simulink model "MPC_MG_raw_ver1"  (R2021b)
settings: Solver=ode23tb  StartTime=0.0  StopTime=1  RelTol=1e-3
model workspace (MAT data in the model file):
  Ts : Simulink.Parameter (value not decoded)
  secondary_on : Simulink.Parameter (value not decoded)
values from neighbouring files (symbols this model uses):
  A = zeros(4,4)    [MPC_MG_script_raw_dmpc.m]    (also in MPG_MG_July.m = [0 1 1 1; 1 0 0 0; 1 0 0 0; 1 0 0 0]; MPG_MG_freq_script.m = ones(4) - eye(4); Script.m = [0 1 1 1 ; 1 0 1 1 ; 1 1 0 1 ; 1 1 1 0])
  a12 = 0    [Four_DG_MG_PrimaryOnlyScript.m]    (also in MPC_MG_script_raw_dmpc.m; MPC_MG_secondary_script.m)
  a14 = 0    [Four_DG_MG_PrimaryOnlyScript.m]    (also in MPC_MG_script_raw_dmpc.m; MPC_MG_secondary_script.m)
  a21 = 1    [Four_DG_MG_PrimaryOnlyScript.m]    (also in MPC_MG_script_raw_dmpc.m; MPC_MG_secondary_script.m)
  a23 = 0    [Four_DG_MG_PrimaryOnlyScript.m]    (also in MPC_MG_script_raw_dmpc.m; MPC_MG_secondary_script.m)
  a32 = 1    [Four_DG_MG_PrimaryOnlyScript.m]    (also in MPC_MG_script_raw_dmpc.m; MPC_MG_secondary_script.m)
  a34 = 0    [Four_DG_MG_PrimaryOnlyScript.m]    (also in MPC_MG_script_raw_dmpc.m; MPC_MG_secondary_script.m)
  a41 = 1    [Four_DG_MG_PrimaryOnlyScript.m]    (also in MPC_MG_script_raw_dmpc.m; MPC_MG_secondary_script.m)
  a43 = 0    [Four_DG_MG_PrimaryOnlyScript.m]    (also in MPC_MG_script_raw_dmpc.m; MPC_MG_secondary_script.m)
  b1v = 1    [Four_DG_MG_PrimaryOnlyScript.m]    (also in MPC_MG_script_raw_dmpc.m; MPC_MG_secondary_script.m; MPG_MG_July.m; MPG_MG_freq_script.m)
  b1w = 1    [Four_DG_MG_PrimaryOnlyScript.m]    (also in MPC_MG_script_raw_dmpc.m; MPC_MG_secondary_script.m; MPG_MG_July.m; MPG_MG_freq_script.m)
  b2v = 0    [Four_DG_MG_PrimaryOnlyScript.m]    (also in MPC_MG_script_raw_dmpc.m; MPC_MG_secondary_script.m; MPG_MG_July.m; MPG_MG_freq_script.m)
  b2w = 0    [Four_DG_MG_PrimaryOnlyScript.m]    (also in MPC_MG_script_raw_dmpc.m; MPC_MG_secondary_script.m; MPG_MG_July.m; MPG_MG_freq_script.m)
  b3v = 0    [Four_DG_MG_PrimaryOnlyScript.m]    (also in MPC_MG_script_raw_dmpc.m; MPC_MG_secondary_script.m; MPG_MG_July.m; MPG_MG_freq_script.m)
  b3w = 0    [Four_DG_MG_PrimaryOnlyScript.m]    (also in MPC_MG_script_raw_dmpc.m; MPC_MG_secondary_script.m; MPG_MG_July.m; MPG_MG_freq_script.m)
  b4v = 0    [Four_DG_MG_PrimaryOnlyScript.m]    (also in MPC_MG_script_raw_dmpc.m; MPC_MG_secondary_script.m; MPG_MG_July.m; MPG_MG_freq_script.m)
  b4w = 0    [Four_DG_MG_PrimaryOnlyScript.m]    (also in MPC_MG_script_raw_dmpc.m; MPC_MG_secondary_script.m; MPG_MG_July.m; MPG_MG_freq_script.m)
  C_f = 50e-6    (= 5e-05)    [Four_DG_MG_PrimaryOnlyScript.m]    (also in MPC_MG_script.m; MPC_MG_script_raw_dmpc.m; MPC_MG_secondary_script.m; MPG_MG_July.m)
  cf = 60    [Four_DG_MG_PrimaryOnlyScript.m]    (also in MPC_MG_script_raw_dmpc.m = 40; MPC_MG_secondary_script.m = 40; MPG_MG_July.m = 100; MPG_MG_freq_script.m = 100)
  cv = 60    [Four_DG_MG_PrimaryOnlyScript.m]    (also in MPC_MG_script_raw_dmpc.m = 40; MPC_MG_secondary_script.m = 40; MPG_MG_July.m = 100; MPG_MG_freq_script.m = 100)
  f_c = 5000    [Four_DG_MG_PrimaryOnlyScript.m]    (also in MPC_MG_script.m = 40000; MPC_MG_script_raw_dmpc.m = 40000; MPC_MG_secondary_script.m = 40000; MPG_MG_July.m = 50000)
  kL = 1e-5    (= 1e-05)    [Four_DG_MG_PrimaryOnlyScript.m]    (also in MPC_MG_script.m = 1e-08; MPC_MG_script_raw_dmpc.m = 1e-08; MPC_MG_secondary_script.m = 1e-07; MPG_MG_July.m = 1e-07)
  L_f = 1.35e-3    (= 0.00135)    [Four_DG_MG_PrimaryOnlyScript.m]    (also in MPC_MG_script.m; MPC_MG_script_raw_dmpc.m; MPC_MG_secondary_script.m; MPG_MG_July.m)
  L_in1 = 0.35e-3    (= 0.00035)    [Four_DG_MG_PrimaryOnlyScript.m]    (also in MPC_MG_script.m; MPC_MG_script_raw_dmpc.m; MPC_MG_secondary_script.m; MPG_MG_July.m)
  L_in2 = 0.35e-3    (= 0.00035)    [Four_DG_MG_PrimaryOnlyScript.m]    (also in MPC_MG_script.m; MPC_MG_script_raw_dmpc.m; MPC_MG_secondary_script.m; MPG_MG_July.m)
  L_in3 = 0.35e-3    (= 0.00035)    [Four_DG_MG_PrimaryOnlyScript.m]    (also in MPC_MG_script.m; MPC_MG_script_raw_dmpc.m; MPC_MG_secondary_script.m; MPG_MG_July.m)
  lambda1 = [30000 50000 90000 50000]'    [MPC_MG_script_raw_dmpc.m]    (also in MPG_MG_July.m = [4 4 4 4]'; MPG_MG_freq_script.m = [3 3 3 3]'; Script.m = [1 1 1 1]')
  lambda2 = [5 6 7 6]'    [MPC_MG_script_raw_dmpc.m]    (also in MPG_MG_July.m = [0.5e-2 0.5e-2 0.5e-2 0.5e-2]'; MPG_MG_freq_script.m = [1.1 1.9 1.5 1.2]'; Script.m = [0.8e-2 0.8e-2 0.8e-2 0.8e-2]')
  lambda3 = [80000 80000 900000 80000]'    [MPC_MG_script_raw_dmpc.m]    (also in MPG_MG_July.m = [1e-3 1e-3 1e-3 1e-3]'; MPG_MG_freq_script.m = [9e-4 1.2e-2 3e-3 3e-3]'; Script.m = [1.5e-3 1.5e-3 1.5e-3 1.5e-3]')
  lambda4 = [5000 5000 5000 5000]'    [MPC_MG_script_raw_dmpc.m]
  lambda5 = [150 130 200 130]'    [MPC_MG_script_raw_dmpc.m]
  lambda6 = [5000 2000 1000 2000]'    [MPC_MG_script_raw_dmpc.m]
  LD_ref1 = 800e-6    (= 0.0008)    [Four_DG_MG_PrimaryOnlyScript.m]    (also in MPC_MG_script.m = 0.0003; MPC_MG_script_raw_dmpc.m = 0.0003; MPC_MG_secondary_script.m = 0.0001; MPG_MG_July.m = 0.0004)
  lo_co = 0.2    [Four_DG_MG_PrimaryOnlyScript.m]    (also in MPC_MG_script.m = 0.05; MPC_MG_script_raw_dmpc.m = 0.1; MPC_MG_secondary_script.m = 0.08; MPG_MG_July.m = 0.15)
  m_p1 = 9.4e-5/droopDivide    (= 9.4e-05)    [Four_DG_MG_PrimaryOnlyScript.m]    (also in MPC_MG_script.m; MPC_MG_script_raw_dmpc.m; MPC_MG_secondary_script.m; MPG_MG_July.m)
  m_p2 = 9.4e-5/droopDivide    (= 9.4e-05)    [Four_DG_MG_PrimaryOnlyScript.m]    (also in MPC_MG_script.m; MPC_MG_script_raw_dmpc.m; MPC_MG_secondary_script.m; MPG_MG_July.m)
  m_p3 = 12.5e-5/droopDivide    (= 0.000125)    [Four_DG_MG_PrimaryOnlyScript.m]    (also in MPC_MG_script.m; MPC_MG_script_raw_dmpc.m; MPC_MG_secondary_script.m; MPG_MG_July.m)
  m_p4 = 12.5e-5/droopDivide    (= 0.000125)    [Four_DG_MG_PrimaryOnlyScript.m]    (also in MPC_MG_script.m; MPC_MG_script_raw_dmpc.m; MPC_MG_secondary_script.m; MPG_MG_July.m)
  n_q1 = 1.3e-3/droopDivide2    (= 0.00013)    [Four_DG_MG_PrimaryOnlyScript.m]    (also in MPC_MG_script.m; MPC_MG_script_raw_dmpc.m; MPC_MG_secondary_script.m; MPG_MG_July.m)
  n_q2 = 1.3e-3/droopDivide2    (= 0.00013)    [Four_DG_MG_PrimaryOnlyScript.m]    (also in MPC_MG_script.m; MPC_MG_script_raw_dmpc.m; MPC_MG_secondary_script.m; MPG_MG_July.m)
  n_q3 = 1.5e-3/droopDivide2    (= 0.00015)    [Four_DG_MG_PrimaryOnlyScript.m]    (also in MPC_MG_script.m; MPC_MG_script_raw_dmpc.m; MPC_MG_secondary_script.m; MPG_MG_July.m)
  n_q4 = 1.5e-3/droopDivide2    (= 0.00015)    [Four_DG_MG_PrimaryOnlyScript.m]    (also in MPC_MG_script.m; MPC_MG_script_raw_dmpc.m; MPC_MG_secondary_script.m; MPG_MG_July.m)
  R_f = 0.1    [Four_DG_MG_PrimaryOnlyScript.m]    (also in MPC_MG_script.m; MPC_MG_script_raw_dmpc.m; MPC_MG_secondary_script.m; MPG_MG_July.m)
  R_in1 = 0.03    [Four_DG_MG_PrimaryOnlyScript.m]    (also in MPC_MG_script.m; MPC_MG_script_raw_dmpc.m; MPC_MG_secondary_script.m; MPG_MG_July.m)
  R_in2 = 0.03    [Four_DG_MG_PrimaryOnlyScript.m]    (also in MPC_MG_script.m; MPC_MG_script_raw_dmpc.m; MPC_MG_secondary_script.m; MPG_MG_July.m)
  R_in3 = 0.03    [Four_DG_MG_PrimaryOnlyScript.m]    (also in MPC_MG_script.m; MPC_MG_script_raw_dmpc.m; MPC_MG_secondary_script.m; MPG_MG_July.m)
  Smax = [45e3 45e3 37e3 37e3]'    [MPC_MG_script_raw_dmpc.m]
  Smax1 = 2400    [MPC_MG_script_raw_dmpc.m]
  Smax2 = 2400    [MPC_MG_script_raw_dmpc.m]
  Smax3 = 2400    [MPC_MG_script_raw_dmpc.m]
  Smax4 = 2400    [MPC_MG_script_raw_dmpc.m]
  time_thresh = 0.6    [Four_DG_MG_PrimaryOnlyScript.m]    (also in MPC_MG_script_raw_dmpc.m = 2; MPC_MG_secondary_script.m = 2; MPG_MG_July.m = 0.5; MPG_MG_freq_script.m = 0.5)
  Ts = 10e-6    (= 1e-05)    [Four_DG_MG_PrimaryOnlyScript.m]    (also in MPC_MG_script.m; MPC_MG_script_raw_dmpc.m; MPC_MG_secondary_script.m; MPG_MG_July.m)
  V_nom = 220*sqrt(2)    [Four_DG_MG_PrimaryOnlyScript.m]    (also in MPC_MG_script.m; MPC_MG_script_raw_dmpc.m; MPC_MG_secondary_script.m; MPG_MG_July.m)
  Vdc = 600    [Four_DG_MG_PrimaryOnlyScript.m]    (also in MPC_MG_script.m; MPC_MG_script_raw_dmpc.m; MPC_MG_secondary_script.m; MPG_MG_July.m)
  Vmax = 155    [MPC_MG_script_raw_dmpc.m]
  Vmin = 145    [MPC_MG_script_raw_dmpc.m]
  w_c_high = 2*pi*50    (= 314.159265359)    [Four_DG_MG_PrimaryOnlyScript.m]    (also in MPC_MG_script.m; MPC_MG_script_raw_dmpc.m; MPC_MG_secondary_script.m; MPG_MG_July.m)
  w_nom = 2*pi*50    (= 314.159265359)    [Four_DG_MG_PrimaryOnlyScript.m]    (also in MPC_MG_script.m; MPC_MG_script_raw_dmpc.m; MPC_MG_secondary_script.m; MPG_MG_July.m)
undefined symbols (not defined in the file or in its folder): i
libraries: spsThreePhaseSeriesRLCBranchLib x18, spsThreePhaseVIMeasurementLib x16, spsabctodq0Lib x16, eeGeneralControl x10, spsPLL3phLib x8, dspswit3 x5, powerlib x5, spsPMUPLLBasedPositiveSequenceLib x4, spsDCVoltageSourceLib x4, spsSeriesRLCBranchLib x4, spsTwoLevelConverterLib x4, spsThreePhaseSeriesRLCLoadLib x3
(part 3 of 4)

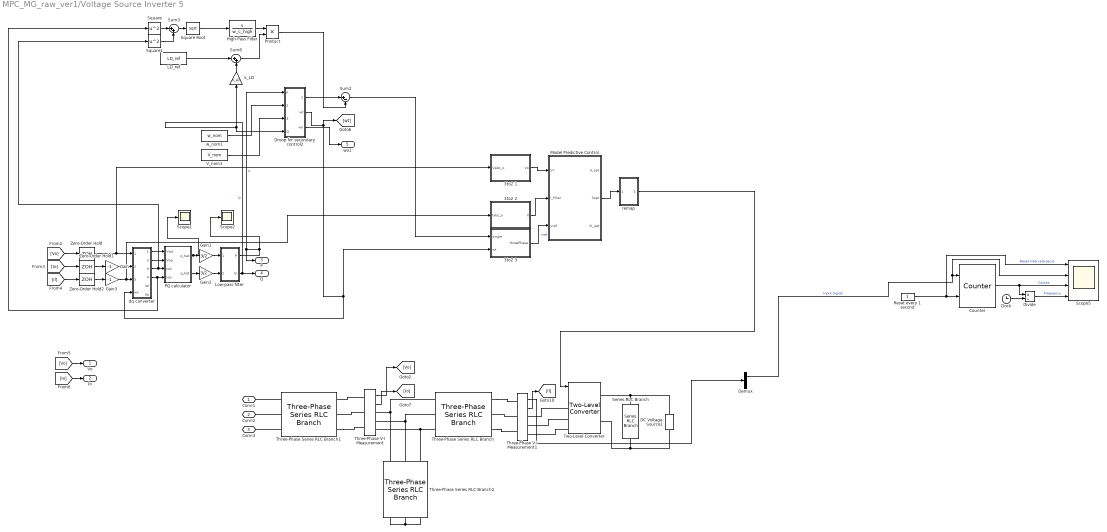
== system MPC_MG_raw_ver1/Voltage Source Inverter 5 ==
  3to2 1 : Subsystem
  3to2 2 : Subsystem
  3to2 3 : Subsystem
  Clock : Clock
  Counter : dspswit3/Counter  Direction=Up  CountEvent=Rising edge  CounterSize=User defined  MaxCount=5e5  InitialCount=0  Output=Count  HitValue=1  ResetInput=on  SamplesPerFrame=1  Ts=1  CntDtype=double  HitDtype=Logical
  DC Voltage Source1 : powerlib/Electrical Sources/DC Voltage Source  Amplitude=Vdc  Measurements=None
  Demux : Demux  Outputs=3
  Divide : Product  Inputs=*/
  Droop for secondary control2 : Subsystem
  Gain : Gain  Gain=-1
  Gain1 : Gain  Gain=3/2
  Gain2 : Gain  Gain=3/2
  Gain3 : Gain  Gain=-1
  High-Pass Filter : TransferFcn  Numerator=[1 0]  Denominator=w_c_high
  LD_ref : Constant  Value=LD_ref
  Low-pass filter : Subsystem
  "Model Predictive Control " : MATLAB Function  TreatAsAtomicUnit=on  mask{Ts=modT, Cfilter=C_f, Lfilter=L_f, Vdc=Vdc}
      mask prompts: Ts "Sampling Time"; Cfilter "Filter Capacitor"; Lfilter "Filter Inductance"; Vdc "Input DC Voltage"
  PQ calculator : Subsystem
  Product : Product
  Reset every 1 second : Constant
  Scope1 : Scope
  Scope2 : Scope
  Scope5 : Scope  NumInputPorts=4
  Series RLC Branch : powerlib/Elements/Series RLC Branch  LConnTagsString=__new0  RConnTagsString=__new0  BranchType=RC  Resistance=30  Inductance=1e-3  SetiL0=off  InitialCurrent=0  Capacitance=80e-6  Setx0=off  InitialVoltage=0  Measurements=None
  Square : Math  Operator=square  SaturateOnIntegerOverflow=on
  Square Root : Sqrt  SaturateOnIntegerOverflow=on
  Square1 : Math  Operator=square  SaturateOnIntegerOverflow=on
  Sum2 : Sum  Inputs=|+-
  Sum3 : Sum  Inputs=|++
  Sum8 : Sum  Inputs=|++
  Three-Phase Series RLC Branch : spsThreePhaseSeriesRLCBranchLib/Three-Phase Series RLC Branch  LConnTagsString=A|B|C  RConnTagsString=A|B|C  BranchType=RL  Resistance=R_f  Inductance=L_f  Capacitance=1e-6  Measurements=None
  Three-Phase Series RLC Branch1 : spsThreePhaseSeriesRLCBranchLib/Three-Phase Series RLC Branch  LConnTagsString=A|B|C  RConnTagsString=A|B|C  BranchType=RL  Resistance=R_in  Inductance=L_in  Capacitance=1e-6  Measurements=None
  Three-Phase Series RLC Branch2 : spsThreePhaseSeriesRLCBranchLib/Three-Phase Series RLC Branch  LConnTagsString=A|B|C  RConnTagsString=A|B|C  BranchType=C  Resistance=R_f  Inductance=1e-3  Capacitance=C_f  Measurements=None
  Three-Phase V-I Measurement : powerlib/Measurements/Three-Phase V-I Measurement  VoltageMeasurement=phase-to-ground  SetLabelV=off  LabelV=Vo1  Vpu=off  VpuLL=off  CurrentMeasurement=yes  SetLabelI=off  LabelI=Io1  Ipu=off  Pbase=100e6  Vbase=500e3  OutputType=Complex  PhasorSimulation=off  PSBequivalent=0
  Three-Phase V-I Measurement1 : powerlib/Measurements/Three-Phase V-I Measurement  VoltageMeasurement=phase-to-ground  SetLabelV=off  LabelV=Vl2  Vpu=off  VpuLL=off  CurrentMeasurement=yes  SetLabelI=off  LabelI=Il2  Ipu=off  Pbase=100e6  Vbase=500e3  OutputType=Complex  PhasorSimulation=off  PSBequivalent=0
  Two-Level Converter : powerlib/Power Electronics/Two-Level Converter  ModelType=Switching devices  Ron=1e-3  Rs=1e6  Cs=inf  Vforward=[0,0]  Ron_Diode=1e-3  Rs_Diode=1e6  Cs_Diode=inf  Vf_Diode=1e-3  Rs_CurrentSource=inf
      settings: SourceProductBaseCode=PS
  V_nom1 : Constant  Value=V_nom
  Zero-Order Hold : ZeroOrderHold  SampleTime=modT
  Zero-Order Hold1 : ZeroOrderHold  SampleTime=modT
  Zero-Order Hold2 : ZeroOrderHold  SampleTime=modT
  dq converter : Subsystem
  k_LD : Gain  Gain=k_LD
  remap : Subsystem
  w_nom1 : Constant  Value=w_nom
  Conn1 : PMIOPort  Side=Left
  Conn2 : PMIOPort  Port=2  Side=Left
  Conn3 : PMIOPort  Port=3  Side=Left
  Vo : Outport
  Io : Outport  Port=2
  P : Outport  Port=3
  Q : Outport  Port=4
  wo1 : Outport  Port=5
  wires:
  Gain/1 -> dq converter/2(Iodq)
  Droop for secondary control2/2(wt) -> [wt], dq converter/4(wo), 3to2 3/2("wt ")
  Gain2/1 -> Low-pass filter/2(q_hat)
  PQ calculator/2(q_hat) -> Gain2/1
  Gain1/1 -> Low-pass filter/1(p_hat)
  dq converter/2(Voq) -> PQ calculator/2(Voq)
  [Il] -> Zero-Order Hold2/1
  PQ calculator/1(p_hat) -> Scope1/1, Gain1/1
  [Io] -> Zero-Order Hold1/1
  dq converter/1(Vod) -> PQ calculator/1(Vod)
  [Vo] -> Vo/1
  [Io] -> Io/1
  Three-Phase V-I Measurement/1 -> [Vo]
  Three-Phase V-I Measurement/2 -> [Io]
  Three-Phase V-I Measurement1/2 -> [Il]
  3to2 1/1(Vo) -> "Model Predictive Control "/1(Vc)
  3to2 3/1(threePhase) -> "Model Predictive Control "/3(vref)  "vref"
  3to2 2/1(Il) -> "Model Predictive Control "/2(i_filter)
  [Vo] -> Zero-Order Hold/1
  "Model Predictive Control "/2(Sopt) -> remap/1(In1)
  Gain3/1 -> 3to2 2/1("Iabc_o "), dq converter/3(Ildq)
  remap/1(Out1) -> Two-Level Converter/1
  Zero-Order Hold/1 -> 3to2 1/1("Vabc_o "), dq converter/1(Vodq)
  Zero-Order Hold1/1 -> Gain/1
  Zero-Order Hold2/1 -> Gain3/1
  Sum2/1 -> 3to2 3/1("single ")
  Three-Phase V-I Measurement1/1 -> Demux/1
  Demux/1 -> Counter/1, Scope5/2  "Input Signal"
  Clock/1 -> Divide/2
  Reset every 1 second/1 -> Scope5/1, Counter/2  "Reset Intervals(secs)"
  Counter/1 -> Scope5/3, Divide/1  "Counts"
  Divide/1 -> Scope5/4  "Frequency"
  w_nom1/1 -> Droop for secondary control2/2(w_nom)
  V_nom1/1 -> Droop for secondary control2/3(V_nom)
  Square1/1 -> Sum3/2
  Sum3/1 -> Square Root/1
  Sum8/1 -> Product/2
  k_LD/1 -> Sum8/2
  Square Root/1 -> High-Pass Filter/1
  Low-pass filter/2(Q) -> Q/1, Droop for secondary control2/4(Q), k_LD/1  "Q"
  Droop for secondary control2/1(Vref) -> Sum2/1
  LD_ref/1 -> Sum8/1
  dq converter/3(Iod) -> Square1/1, PQ calculator/3(Iod)
  Droop for secondary control2/3(wo) -> wo1/1
  Product/1 -> Sum2/2
  dq converter/4(Ioq) -> Square/1, PQ calculator/4(Ioq)
  High-Pass Filter/1 -> Product/1
  Low-pass filter/1(P) -> Scope2/1, P/1, Droop for secondary control2/1(P)  "P"
  Square/1 -> Sum3/1
  connections:
  Three-Phase Series RLC Branch2/LConn1 -- Three-Phase V-I Measurement/RConn1 -- Three-Phase Series RLC Branch/LConn1
  Two-Level Converter/RConn1 -- DC Voltage Source1/RConn1 -- Series RLC Branch/LConn1
  Three-Phase Series RLC Branch2/RConn3 -- Three-Phase Series RLC Branch2/RConn1 -- Three-Phase Series RLC Branch2/RConn2
  Three-Phase Series RLC Branch2/LConn3 -- Three-Phase Series RLC Branch/LConn3 -- Three-Phase V-I Measurement/RConn3
  Two-Level Converter/RConn2 -- Series RLC Branch/RConn1 -- DC Voltage Source1/LConn1
  Three-Phase Series RLC Branch/LConn2 -- Three-Phase V-I Measurement/RConn2 -- Three-Phase Series RLC Branch2/LConn2
  Two-Level Converter/LConn1 -- Three-Phase V-I Measurement1/RConn1
  Three-Phase V-I Measurement1/LConn2 -- Three-Phase Series RLC Branch/RConn2
  Two-Level Converter/LConn2 -- Three-Phase V-I Measurement1/RConn2
  Three-Phase Series RLC Branch1/LConn2 -- Conn2/RConn1
  Two-Level Converter/LConn3 -- Three-Phase V-I Measurement1/RConn3
  Three-Phase Series RLC Branch/RConn1 -- Three-Phase V-I Measurement1/LConn1
  Three-Phase Series RLC Branch1/LConn3 -- Conn3/RConn1
  Three-Phase V-I Measurement/LConn1 -- Three-Phase Series RLC Branch1/RConn1
  Three-Phase Series RLC Branch1/LConn1 -- Conn1/RConn1
  Three-Phase V-I Measurement/LConn2 -- Three-Phase Series RLC Branch1/RConn2
  Three-Phase Series RLC Branch1/RConn3 -- Three-Phase V-I Measurement/LConn3
  Three-Phase Series RLC Branch/RConn3 -- Three-Phase V-I Measurement1/LConn3

== system MPC_MG_raw_ver1/Voltage Source Inverter 1/3to2 1 ==
  "Vabc_o " : Inport
  Add : Sum  Inputs=+++
  Constant : Constant  Value=exp(i*2*pi/3)
  Constant1 : Constant  Value=2/3
  Demux : Demux  Outputs=3
  Math Function : Math  Operator=square  SignedPower=on  SaturateOnIntegerOverflow=on
  Product : Product  RndMeth=Zero
  Product1 : Product  RndMeth=Zero
  Product2 : Product  RndMeth=Zero
  Vo : Outport  VectorParamsAs1DForOutWhenUnconnected=off
  wires:
  Add/1 -> Product/1
  Demux/1 -> Add/1
  Constant1/1 -> Product/2
  Product1/1 -> Add/2
  Constant/1 -> Product1/1, Math Function/1
  Demux/2 -> Product1/2
  Math Function/1 -> Product2/1
  Demux/3 -> Product2/2
  Product2/1 -> Add/3
  Product/1 -> Vo/1
  "Vabc_o "/1 -> Demux/1

== system MPC_MG_raw_ver1/Voltage Source Inverter 1/3to2 2 ==
  "Iabc_o " : Inport
  Add : Sum  Inputs=+++
  Constant : Constant  Value=exp(i*2*pi/3)
  Constant1 : Constant  Value=2/3
  Demux : Demux  Outputs=3
  Math Function : Math  Operator=square  SignedPower=on  SaturateOnIntegerOverflow=on
  Product : Product  RndMeth=Zero
  Product1 : Product  RndMeth=Zero
  Product2 : Product  RndMeth=Zero
  Il : Outport  VectorParamsAs1DForOutWhenUnconnected=off
  wires:
  Add/1 -> Product/1
  Demux/1 -> Add/1
  Constant1/1 -> Product/2
  Product1/1 -> Add/2
  Constant/1 -> Product1/1, Math Function/1
  Demux/2 -> Product1/2
  Math Function/1 -> Product2/1
  Demux/3 -> Product2/2
  Product2/1 -> Add/3
  Product/1 -> Il/1
  "Iabc_o "/1 -> Demux/1

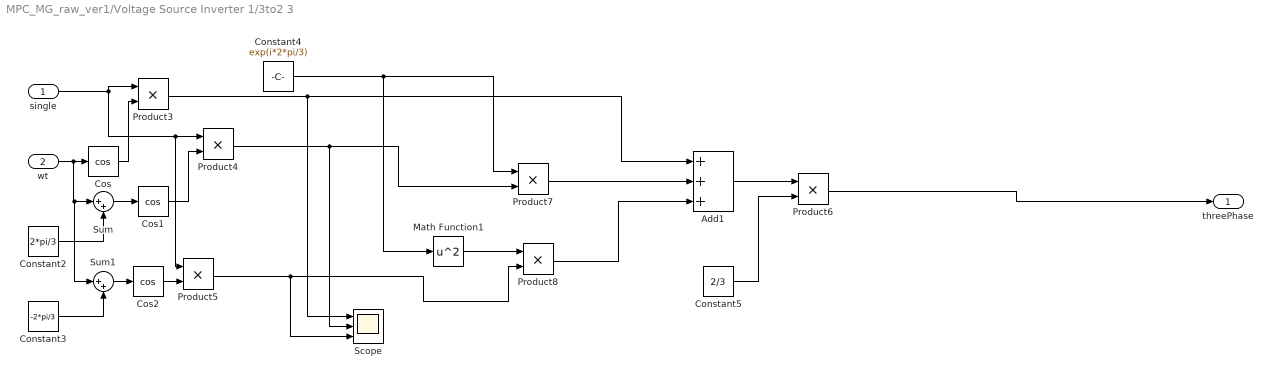
== system MPC_MG_raw_ver1/Voltage Source Inverter 1/3to2 3 ==
  "single " : Inport
  "wt " : Inport  Port=2
  Add1 : Sum  Inputs=+++
  Constant2 : Constant  Value=2*pi/3
  Constant3 : Constant  Value=-2*pi/3
  Constant4 : Constant  Value=exp(i*2*pi/3)
  Constant5 : Constant  Value=2/3
  Cos : Trigonometry  Operator=cos
  Cos1 : Trigonometry  Operator=cos
  Cos2 : Trigonometry  Operator=cos
  Math Function1 : Math  Operator=square  SignedPower=on  SaturateOnIntegerOverflow=on
  Product{3..8} (6 alike) : Product  RndMeth=Zero
  Scope : Scope  NumInputPorts=3
  Sum : Sum  Inputs=|++
  Sum1 : Sum  Inputs=|++
  threePhase : Outport  VectorParamsAs1DForOutWhenUnconnected=off
  wires:
  "single "/1 -> Product5/1, Product4/1, Product3/1
  Cos/1 -> Product3/2
  Constant2/1 -> Sum/2
  Sum/1 -> Cos1/1
  Cos1/1 -> Product4/2
  "wt "/1 -> Sum1/1, Sum/1, Cos/1
  Constant3/1 -> Sum1/2
  Sum1/1 -> Cos2/1
  Cos2/1 -> Product5/2
  Constant4/1 -> Product7/1, Math Function1/1
  Product7/1 -> Add1/2
  Add1/1 -> Product6/1
  Product8/1 -> Add1/3
  Product5/1 -> Scope/3, Product8/2
  Product6/1 -> threePhase/1
  Product3/1 -> Scope/1, Add1/1
  Constant5/1 -> Product6/2
  Product4/1 -> Scope/2, Product7/2
  Math Function1/1 -> Product8/1

== system MPC_MG_raw_ver1/Voltage Source Inverter 1/Droop for secondary control2 ==
  P : Inport
  w_nom : Inport  Port=2
  V_nom : Inport  Port=3
  Q : Inport  Port=4
  Gain4 : Gain  Gain=n_q
  Gain5 : Gain  Gain=m_p
  Integrator : Integrator  WrapState=on  WrappedStateUpperValue=2*pi  WrappedStateLowerValue=0
  Sum1 : Sum  Inputs=|+-
  Sum2 : Sum  Inputs=|+-
  Vref : Outport
  wt : Outport  Port=2
  wo : Outport  Port=3
  wires:
  P/1 -> Gain5/1
  w_nom/1 -> Sum2/1
  Gain5/1 -> Sum2/2
  Sum2/1 -> wo/1, Integrator/1  "w"
  Integrator/1 -> wt/1
  V_nom/1 -> Sum1/1  "Vod_s"
  Gain4/1 -> Sum1/2
  Q/1 -> Gain4/1
  Sum1/1 -> Vref/1  "Vod_s"

== system MPC_MG_raw_ver1/Voltage Source Inverter 1/Low-pass filter ==
  p_hat : Inport
  q_hat : Inport  Port=2
  Low-Pass Filter (Discrete or Continuous) : eeGeneralControl/Low-Pass Filter (Discrete or Continuous)  K=1  T=lo_co  B=inf  A=-inf  init_option=Inherited from block input  x0=0  Ts=-1
  Low-Pass Filter (Discrete or Continuous)1 : eeGeneralControl/Low-Pass Filter (Discrete or Continuous)  K=1  T=lo_co  B=inf  A=-inf  init_option=Inherited from block input  x0=0  Ts=-1
  P : Outport
  Q : Outport  Port=2
  wires:
  q_hat/1 -> Low-Pass Filter (Discrete or Continuous)1/1
  Low-Pass Filter (Discrete or Continuous)1/1 -> Q/1  "Q"
  Low-Pass Filter (Discrete or Continuous)/1 -> P/1  "P"
  p_hat/1 -> Low-Pass Filter (Discrete or Continuous)/1

== system MPC_MG_raw_ver1/Voltage Source Inverter 1/PQ calculator ==
  Vod : Inport
  Voq : Inport  Port=2
  Iod : Inport  Port=3
  Ioq : Inport  Port=4
  Product{,1..3} (4 alike) : Product
  Sum10 : Sum  Inputs=|++
  Sum11 : Sum  Inputs=|+-
  p_hat : Outport
  q_hat : Outport  Port=2
  wires:
  Product3/1 -> Sum11/2
  Product1/1 -> Sum10/2
  Voq/1 -> Product3/1, Product1/1
  Iod/1 -> Product/2, Product3/2
  Product2/1 -> Sum11/1
  Ioq/1 -> Product1/2, Product2/2
  Product/1 -> Sum10/1
  Vod/1 -> Product/1, Product2/1
  Sum11/1 -> q_hat/1  "q_hat"
  Sum10/1 -> p_hat/1  "p_hat"

== system MPC_MG_raw_ver1/Voltage Source Inverter 1/dq converter ==
  Vodq : Inport
  Iodq : Inport  Port=2
  Ildq : Inport  Port=3
  wo : Inport  Port=4
  Demux : Demux  Outputs=2
  Demux1 : Demux  Outputs=2
  Demux4 : Demux  Outputs=2
  Selector1 : Selector  InputPortWidth=3  IndexOptions=Index vector (dialog)  Indices=[1 2]  OutputSizes=1
  Selector2 : Selector  InputPortWidth=3  IndexOptions=Index vector (dialog)  Indices=[1 2]  OutputSizes=1
  Selector3 : Selector  InputPortWidth=3  IndexOptions=Index vector (dialog)  Indices=[1 2]  OutputSizes=1
  abc to dq0 : spsabctodq0Lib/abc to dq0  Alignment=90 degrees behind phase A axis
  abc to dq1 : spsabctodq0Lib/abc to dq0  Alignment=90 degrees behind phase A axis
  abc to dq2 : spsabctodq0Lib/abc to dq0  Alignment=90 degrees behind phase A axis
  Vod : Outport
  Voq : Outport  Port=2
  Iod : Outport  Port=3
  Ioq : Outport  Port=4
  Ild : Outport  Port=5
  Ilq : Outport  Port=6
  wires:
  Vodq/1 -> abc to dq0/1
  Demux/1 -> Vod/1  "Vod"
  Demux1/1 -> Iod/1  "Iod"
  Selector3/1 -> Demux4/1
  Demux/2 -> Voq/1  "Voq"
  Selector1/1 -> Demux/1
  abc to dq2/1 -> Selector2/1
  abc to dq1/1 -> Selector3/1
  wo/1 -> abc to dq0/2, abc to dq2/2, abc to dq1/2
  Demux1/2 -> Ioq/1  "Ioq"
  Demux4/1 -> Ild/1  "Ild"
  abc to dq0/1 -> Selector1/1
  Selector2/1 -> Demux1/1
  Iodq/1 -> abc to dq2/1
  Ildq/1 -> abc to dq1/1
  Demux4/2 -> Ilq/1  "Ilq"

== system MPC_MG_raw_ver1/Voltage Source Inverter 1/remap ==
  In1 : Inport
  Demux : Demux  Outputs=6
  Mux : Mux  Inputs=6
  Out1 : Outport
  wires:
  Demux/5 -> Mux/4
  Demux/3 -> Mux/5
  Demux/2 -> Mux/3
  Demux/4 -> Mux/2
  In1/1 -> Demux/1
  Demux/1 -> Mux/1
  Demux/6 -> Mux/6
  Mux/1 -> Out1/1

== system MPC_MG_raw_ver1/Voltage Source Inverter 2/3to2 1 ==
  "Vabc_o " : Inport
  Add : Sum  Inputs=+++
  Constant : Constant  Value=exp(i*2*pi/3)
  Constant1 : Constant  Value=2/3
  Demux : Demux  Outputs=3
  Math Function : Math  Operator=square  SignedPower=on  SaturateOnIntegerOverflow=on
  Product : Product  RndMeth=Zero
  Product1 : Product  RndMeth=Zero
  Product2 : Product  RndMeth=Zero
  Vo : Outport  VectorParamsAs1DForOutWhenUnconnected=off
  wires:
  Add/1 -> Product/1
  Demux/1 -> Add/1
  Constant1/1 -> Product/2
  Product1/1 -> Add/2
  Constant/1 -> Product1/1, Math Function/1
  Demux/2 -> Product1/2
  Math Function/1 -> Product2/1
  Demux/3 -> Product2/2
  Product2/1 -> Add/3
  Product/1 -> Vo/1
  "Vabc_o "/1 -> Demux/1

== system MPC_MG_raw_ver1/Voltage Source Inverter 2/3to2 2 ==
  "Iabc_o " : Inport
  Add : Sum  Inputs=+++
  Constant : Constant  Value=exp(i*2*pi/3)
  Constant1 : Constant  Value=2/3
  Demux : Demux  Outputs=3
  Math Function : Math  Operator=square  SignedPower=on  SaturateOnIntegerOverflow=on
  Product : Product  RndMeth=Zero
  Product1 : Product  RndMeth=Zero
  Product2 : Product  RndMeth=Zero
  Il : Outport  VectorParamsAs1DForOutWhenUnconnected=off
  wires:
  Add/1 -> Product/1
  Demux/1 -> Add/1
  Constant1/1 -> Product/2
  Product1/1 -> Add/2
  Constant/1 -> Product1/1, Math Function/1
  Demux/2 -> Product1/2
  Math Function/1 -> Product2/1
  Demux/3 -> Product2/2
  Product2/1 -> Add/3
  Product/1 -> Il/1
  "Iabc_o "/1 -> Demux/1

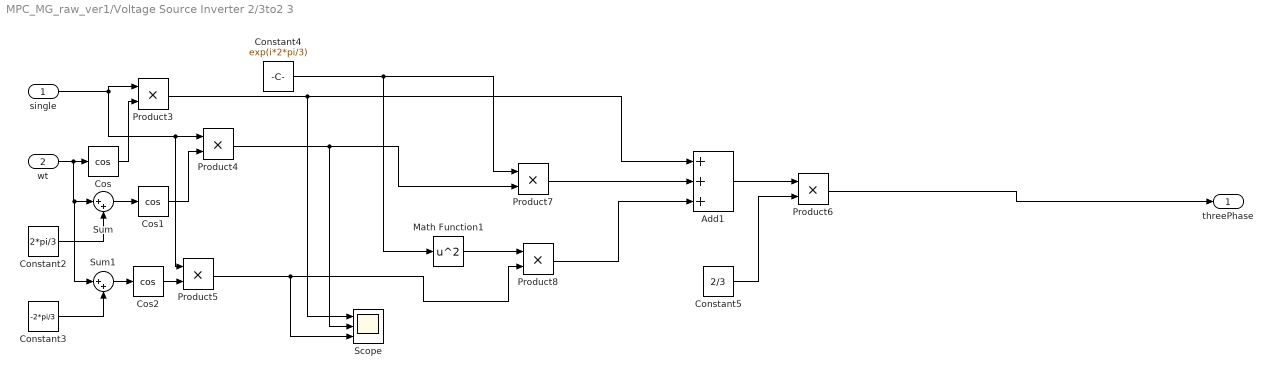
== system MPC_MG_raw_ver1/Voltage Source Inverter 2/3to2 3 ==
  "single " : Inport
  "wt " : Inport  Port=2
  Add1 : Sum  Inputs=+++
  Constant2 : Constant  Value=2*pi/3
  Constant3 : Constant  Value=-2*pi/3
  Constant4 : Constant  Value=exp(i*2*pi/3)
  Constant5 : Constant  Value=2/3
  Cos : Trigonometry  Operator=cos
  Cos1 : Trigonometry  Operator=cos
  Cos2 : Trigonometry  Operator=cos
  Math Function1 : Math  Operator=square  SignedPower=on  SaturateOnIntegerOverflow=on
  Product{3..8} (6 alike) : Product  RndMeth=Zero
  Scope : Scope  NumInputPorts=3
  Sum : Sum  Inputs=|++
  Sum1 : Sum  Inputs=|++
  threePhase : Outport  VectorParamsAs1DForOutWhenUnconnected=off
  wires:
  "single "/1 -> Product5/1, Product4/1, Product3/1
  Cos/1 -> Product3/2
  Constant2/1 -> Sum/2
  Sum/1 -> Cos1/1
  Cos1/1 -> Product4/2
  "wt "/1 -> Sum1/1, Sum/1, Cos/1
  Constant3/1 -> Sum1/2
  Sum1/1 -> Cos2/1
  Cos2/1 -> Product5/2
  Constant4/1 -> Product7/1, Math Function1/1
  Product7/1 -> Add1/2
  Add1/1 -> Product6/1
  Product8/1 -> Add1/3
  Product5/1 -> Scope/3, Product8/2
  Product6/1 -> threePhase/1
  Product3/1 -> Scope/1, Add1/1
  Constant5/1 -> Product6/2
  Product4/1 -> Scope/2, Product7/2
  Math Function1/1 -> Product8/1

== system MPC_MG_raw_ver1/Voltage Source Inverter 2/Droop for secondary control2 ==
  P : Inport
  w_nom : Inport  Port=2
  V_nom : Inport  Port=3
  Q : Inport  Port=4
  Gain4 : Gain  Gain=n_q
  Gain5 : Gain  Gain=m_p
  Integrator : Integrator  WrapState=on  WrappedStateUpperValue=2*pi  WrappedStateLowerValue=0
  Sum1 : Sum  Inputs=|+-
  Sum2 : Sum  Inputs=|+-
  Vref : Outport
  wt : Outport  Port=2
  wo : Outport  Port=3
  wires:
  P/1 -> Gain5/1
  w_nom/1 -> Sum2/1
  Gain5/1 -> Sum2/2
  Sum2/1 -> wo/1, Integrator/1  "w"
  Integrator/1 -> wt/1
  V_nom/1 -> Sum1/1  "Vod_s"
  Gain4/1 -> Sum1/2
  Q/1 -> Gain4/1
  Sum1/1 -> Vref/1  "Vod_s"

== system MPC_MG_raw_ver1/Voltage Source Inverter 2/Low-pass filter ==
  p_hat : Inport
  q_hat : Inport  Port=2
  Low-Pass Filter (Discrete or Continuous) : eeGeneralControl/Low-Pass Filter (Discrete or Continuous)  K=1  T=lo_co  B=inf  A=-inf  init_option=Inherited from block input  x0=0  Ts=-1
  Low-Pass Filter (Discrete or Continuous)1 : eeGeneralControl/Low-Pass Filter (Discrete or Continuous)  K=1  T=lo_co  B=inf  A=-inf  init_option=Inherited from block input  x0=0  Ts=-1
  P : Outport
  Q : Outport  Port=2
  wires:
  q_hat/1 -> Low-Pass Filter (Discrete or Continuous)1/1
  Low-Pass Filter (Discrete or Continuous)1/1 -> Q/1  "Q"
  Low-Pass Filter (Discrete or Continuous)/1 -> P/1  "P"
  p_hat/1 -> Low-Pass Filter (Discrete or Continuous)/1

== system MPC_MG_raw_ver1/Voltage Source Inverter 2/PQ calculator ==
  Vod : Inport
  Voq : Inport  Port=2
  Iod : Inport  Port=3
  Ioq : Inport  Port=4
  Product{,1..3} (4 alike) : Product
  Sum10 : Sum  Inputs=|++
  Sum11 : Sum  Inputs=|+-
  p_hat : Outport
  q_hat : Outport  Port=2
  wires:
  Product3/1 -> Sum11/2
  Product1/1 -> Sum10/2
  Voq/1 -> Product3/1, Product1/1
  Iod/1 -> Product/2, Product3/2
  Product2/1 -> Sum11/1
  Ioq/1 -> Product1/2, Product2/2
  Product/1 -> Sum10/1
  Vod/1 -> Product/1, Product2/1
  Sum11/1 -> q_hat/1  "q_hat"
  Sum10/1 -> p_hat/1  "p_hat"

== system MPC_MG_raw_ver1/Voltage Source Inverter 2/dq converter ==
  Vodq : Inport
  Iodq : Inport  Port=2
  Ildq : Inport  Port=3
  wo : Inport  Port=4
  Demux : Demux  Outputs=2
  Demux1 : Demux  Outputs=2
  Demux4 : Demux  Outputs=2
  Selector1 : Selector  InputPortWidth=3  IndexOptions=Index vector (dialog)  Indices=[1 2]  OutputSizes=1
  Selector2 : Selector  InputPortWidth=3  IndexOptions=Index vector (dialog)  Indices=[1 2]  OutputSizes=1
  Selector3 : Selector  InputPortWidth=3  IndexOptions=Index vector (dialog)  Indices=[1 2]  OutputSizes=1
  abc to dq0 : spsabctodq0Lib/abc to dq0  Alignment=90 degrees behind phase A axis
  abc to dq1 : spsabctodq0Lib/abc to dq0  Alignment=90 degrees behind phase A axis
  abc to dq2 : spsabctodq0Lib/abc to dq0  Alignment=90 degrees behind phase A axis
  Vod : Outport
  Voq : Outport  Port=2
  Iod : Outport  Port=3
  Ioq : Outport  Port=4
  Ild : Outport  Port=5
  Ilq : Outport  Port=6
  wires:
  Vodq/1 -> abc to dq0/1
  Demux/1 -> Vod/1  "Vod"
  Demux1/1 -> Iod/1  "Iod"
  Selector3/1 -> Demux4/1
  Demux/2 -> Voq/1  "Voq"
  Selector1/1 -> Demux/1
  abc to dq2/1 -> Selector2/1
  abc to dq1/1 -> Selector3/1
  wo/1 -> abc to dq0/2, abc to dq2/2, abc to dq1/2
  Demux1/2 -> Ioq/1  "Ioq"
  Demux4/1 -> Ild/1  "Ild"
  abc to dq0/1 -> Selector1/1
  Selector2/1 -> Demux1/1
  Iodq/1 -> abc to dq2/1
  Ildq/1 -> abc to dq1/1
  Demux4/2 -> Ilq/1  "Ilq"

== system MPC_MG_raw_ver1/Voltage Source Inverter 2/remap ==
  In1 : Inport
  Demux : Demux  Outputs=6
  Mux : Mux  Inputs=6
  Out1 : Outport
  wires:
  Demux/5 -> Mux/4
  Demux/3 -> Mux/5
  Demux/2 -> Mux/3
  Demux/4 -> Mux/2
  In1/1 -> Demux/1
  Demux/1 -> Mux/1
  Demux/6 -> Mux/6
  Mux/1 -> Out1/1

== system MPC_MG_raw_ver1/Voltage Source Inverter 3/3to2 1 ==
  "Vabc_o " : Inport
  Add : Sum  Inputs=+++
  Constant : Constant  Value=exp(i*2*pi/3)
  Constant1 : Constant  Value=2/3
  Demux : Demux  Outputs=3
  Math Function : Math  Operator=square  SignedPower=on  SaturateOnIntegerOverflow=on
  Product : Product  RndMeth=Zero
  Product1 : Product  RndMeth=Zero
  Product2 : Product  RndMeth=Zero
  Vo : Outport  VectorParamsAs1DForOutWhenUnconnected=off
  wires:
  Add/1 -> Product/1
  Demux/1 -> Add/1
  Constant1/1 -> Product/2
  Product1/1 -> Add/2
  Constant/1 -> Product1/1, Math Function/1
  Demux/2 -> Product1/2
  Math Function/1 -> Product2/1
  Demux/3 -> Product2/2
  Product2/1 -> Add/3
  Product/1 -> Vo/1
  "Vabc_o "/1 -> Demux/1

== system MPC_MG_raw_ver1/Voltage Source Inverter 3/3to2 2 ==
  "Iabc_o " : Inport
  Add : Sum  Inputs=+++
  Constant : Constant  Value=exp(i*2*pi/3)
  Constant1 : Constant  Value=2/3
  Demux : Demux  Outputs=3
  Math Function : Math  Operator=square  SignedPower=on  SaturateOnIntegerOverflow=on
  Product : Product  RndMeth=Zero
  Product1 : Product  RndMeth=Zero
  Product2 : Product  RndMeth=Zero
  Il : Outport  VectorParamsAs1DForOutWhenUnconnected=off
  wires:
  Add/1 -> Product/1
  Demux/1 -> Add/1
  Constant1/1 -> Product/2
  Product1/1 -> Add/2
  Constant/1 -> Product1/1, Math Function/1
  Demux/2 -> Product1/2
  Math Function/1 -> Product2/1
  Demux/3 -> Product2/2
  Product2/1 -> Add/3
  Product/1 -> Il/1
  "Iabc_o "/1 -> Demux/1

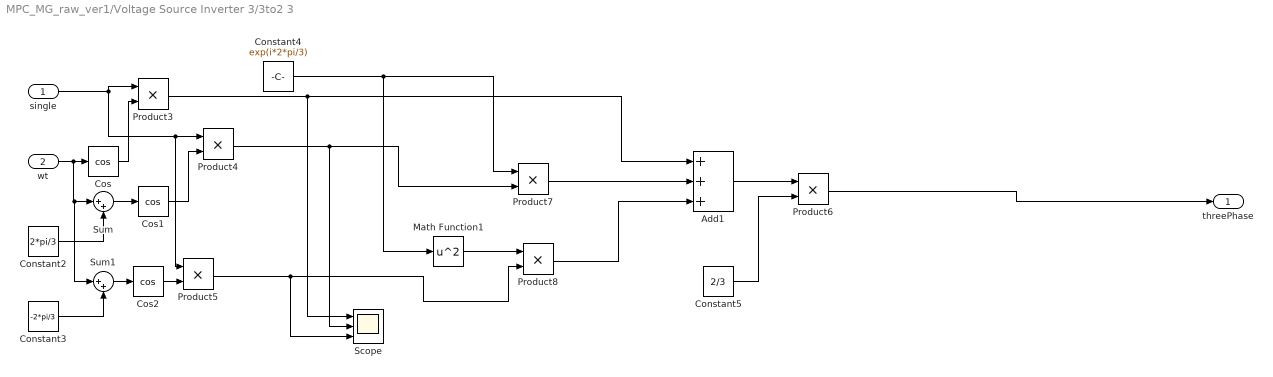
== system MPC_MG_raw_ver1/Voltage Source Inverter 3/3to2 3 ==
  "single " : Inport
  "wt " : Inport  Port=2
  Add1 : Sum  Inputs=+++
  Constant2 : Constant  Value=2*pi/3
  Constant3 : Constant  Value=-2*pi/3
  Constant4 : Constant  Value=exp(i*2*pi/3)
  Constant5 : Constant  Value=2/3
  Cos : Trigonometry  Operator=cos
  Cos1 : Trigonometry  Operator=cos
  Cos2 : Trigonometry  Operator=cos
  Math Function1 : Math  Operator=square  SignedPower=on  SaturateOnIntegerOverflow=on
  Product{3..8} (6 alike) : Product  RndMeth=Zero
  Scope : Scope  NumInputPorts=3
  Sum : Sum  Inputs=|++
  Sum1 : Sum  Inputs=|++
  threePhase : Outport  VectorParamsAs1DForOutWhenUnconnected=off
  wires:
  "single "/1 -> Product5/1, Product4/1, Product3/1
  Cos/1 -> Product3/2
  Constant2/1 -> Sum/2
  Sum/1 -> Cos1/1
  Cos1/1 -> Product4/2
  "wt "/1 -> Sum1/1, Sum/1, Cos/1
  Constant3/1 -> Sum1/2
  Sum1/1 -> Cos2/1
  Cos2/1 -> Product5/2
  Constant4/1 -> Product7/1, Math Function1/1
  Product7/1 -> Add1/2
  Add1/1 -> Product6/1
  Product8/1 -> Add1/3
  Product5/1 -> Scope/3, Product8/2
  Product6/1 -> threePhase/1
  Product3/1 -> Scope/1, Add1/1
  Constant5/1 -> Product6/2
  Product4/1 -> Scope/2, Product7/2
  Math Function1/1 -> Product8/1

== system MPC_MG_raw_ver1/Voltage Source Inverter 3/Droop for secondary control2 ==
  P : Inport
  w_nom : Inport  Port=2
  V_nom : Inport  Port=3
  Q : Inport  Port=4
  Gain4 : Gain  Gain=n_q
  Gain5 : Gain  Gain=m_p
  Integrator : Integrator  WrapState=on  WrappedStateUpperValue=2*pi  WrappedStateLowerValue=0
  Sum1 : Sum  Inputs=|+-
  Sum2 : Sum  Inputs=|+-
  Vref : Outport
  wt : Outport  Port=2
  wo : Outport  Port=3
  wires:
  P/1 -> Gain5/1
  w_nom/1 -> Sum2/1
  Gain5/1 -> Sum2/2
  Sum2/1 -> wo/1, Integrator/1  "w"
  Integrator/1 -> wt/1
  V_nom/1 -> Sum1/1  "Vod_s"
  Gain4/1 -> Sum1/2
  Q/1 -> Gain4/1
  Sum1/1 -> Vref/1  "Vod_s"

== system MPC_MG_raw_ver1/Voltage Source Inverter 3/Low-pass filter ==
  p_hat : Inport
  q_hat : Inport  Port=2
  Low-Pass Filter (Discrete or Continuous) : eeGeneralControl/Low-Pass Filter (Discrete or Continuous)  K=1  T=lo_co  B=inf  A=-inf  init_option=Inherited from block input  x0=0  Ts=-1
  Low-Pass Filter (Discrete or Continuous)1 : eeGeneralControl/Low-Pass Filter (Discrete or Continuous)  K=1  T=lo_co  B=inf  A=-inf  init_option=Inherited from block input  x0=0  Ts=-1
  P : Outport
  Q : Outport  Port=2
  wires:
  q_hat/1 -> Low-Pass Filter (Discrete or Continuous)1/1
  Low-Pass Filter (Discrete or Continuous)1/1 -> Q/1  "Q"
  Low-Pass Filter (Discrete or Continuous)/1 -> P/1  "P"
  p_hat/1 -> Low-Pass Filter (Discrete or Continuous)/1

== system MPC_MG_raw_ver1/Voltage Source Inverter 3/PQ calculator ==
  Vod : Inport
  Voq : Inport  Port=2
  Iod : Inport  Port=3
  Ioq : Inport  Port=4
  Product{,1..3} (4 alike) : Product
  Sum10 : Sum  Inputs=|++
  Sum11 : Sum  Inputs=|+-
  p_hat : Outport
  q_hat : Outport  Port=2
  wires:
  Product3/1 -> Sum11/2
  Product1/1 -> Sum10/2
  Voq/1 -> Product3/1, Product1/1
  Iod/1 -> Product/2, Product3/2
  Product2/1 -> Sum11/1
  Ioq/1 -> Product1/2, Product2/2
  Product/1 -> Sum10/1
  Vod/1 -> Product/1, Product2/1
  Sum11/1 -> q_hat/1  "q_hat"
  Sum10/1 -> p_hat/1  "p_hat"

== system MPC_MG_raw_ver1/Voltage Source Inverter 3/dq converter ==
  Vodq : Inport
  Iodq : Inport  Port=2
  Ildq : Inport  Port=3
  wo : Inport  Port=4
  Demux : Demux  Outputs=2
  Demux1 : Demux  Outputs=2
  Demux4 : Demux  Outputs=2
  Selector1 : Selector  InputPortWidth=3  IndexOptions=Index vector (dialog)  Indices=[1 2]  OutputSizes=1
  Selector2 : Selector  InputPortWidth=3  IndexOptions=Index vector (dialog)  Indices=[1 2]  OutputSizes=1
  Selector3 : Selector  InputPortWidth=3  IndexOptions=Index vector (dialog)  Indices=[1 2]  OutputSizes=1
  abc to dq0 : spsabctodq0Lib/abc to dq0  Alignment=90 degrees behind phase A axis
  abc to dq1 : spsabctodq0Lib/abc to dq0  Alignment=90 degrees behind phase A axis
  abc to dq2 : spsabctodq0Lib/abc to dq0  Alignment=90 degrees behind phase A axis
  Vod : Outport
  Voq : Outport  Port=2
  Iod : Outport  Port=3
  Ioq : Outport  Port=4
  Ild : Outport  Port=5
  Ilq : Outport  Port=6
  wires:
  Vodq/1 -> abc to dq0/1
  Demux/1 -> Vod/1  "Vod"
  Demux1/1 -> Iod/1  "Iod"
  Selector3/1 -> Demux4/1
  Demux/2 -> Voq/1  "Voq"
  Selector1/1 -> Demux/1
  abc to dq2/1 -> Selector2/1
  abc to dq1/1 -> Selector3/1
  wo/1 -> abc to dq0/2, abc to dq2/2, abc to dq1/2
  Demux1/2 -> Ioq/1  "Ioq"
  Demux4/1 -> Ild/1  "Ild"
  abc to dq0/1 -> Selector1/1
  Selector2/1 -> Demux1/1
  Iodq/1 -> abc to dq2/1
  Ildq/1 -> abc to dq1/1
  Demux4/2 -> Ilq/1  "Ilq"

== system MPC_MG_raw_ver1/Voltage Source Inverter 3/remap ==
  In1 : Inport
  Demux : Demux  Outputs=6
  Mux : Mux  Inputs=6
  Out1 : Outport
  wires:
  Demux/5 -> Mux/4
  Demux/3 -> Mux/5
  Demux/2 -> Mux/3
  Demux/4 -> Mux/2
  In1/1 -> Demux/1
  Demux/1 -> Mux/1
  Demux/6 -> Mux/6
  Mux/1 -> Out1/1

== system MPC_MG_raw_ver1/Voltage Source Inverter 4/3to2 1 ==
  "Vabc_o " : Inport
  Add : Sum  Inputs=+++
  Constant : Constant  Value=exp(i*2*pi/3)
  Constant1 : Constant  Value=2/3
  Demux : Demux  Outputs=3
  Math Function : Math  Operator=square  SignedPower=on  SaturateOnIntegerOverflow=on
  Product : Product  RndMeth=Zero
  Product1 : Product  RndMeth=Zero
  Product2 : Product  RndMeth=Zero
  Vo : Outport  VectorParamsAs1DForOutWhenUnconnected=off
  wires:
  Add/1 -> Product/1
  Demux/1 -> Add/1
  Constant1/1 -> Product/2
  Product1/1 -> Add/2
  Constant/1 -> Product1/1, Math Function/1
  Demux/2 -> Product1/2
  Math Function/1 -> Product2/1
  Demux/3 -> Product2/2
  Product2/1 -> Add/3
  Product/1 -> Vo/1
  "Vabc_o "/1 -> Demux/1

== system MPC_MG_raw_ver1/Voltage Source Inverter 4/3to2 2 ==
  "Iabc_o " : Inport
  Add : Sum  Inputs=+++
  Constant : Constant  Value=exp(i*2*pi/3)
  Constant1 : Constant  Value=2/3
  Demux : Demux  Outputs=3
  Math Function : Math  Operator=square  SignedPower=on  SaturateOnIntegerOverflow=on
  Product : Product  RndMeth=Zero
  Product1 : Product  RndMeth=Zero
  Product2 : Product  RndMeth=Zero
  Il : Outport  VectorParamsAs1DForOutWhenUnconnected=off
  wires:
  Add/1 -> Product/1
  Demux/1 -> Add/1
  Constant1/1 -> Product/2
  Product1/1 -> Add/2
  Constant/1 -> Product1/1, Math Function/1
  Demux/2 -> Product1/2
  Math Function/1 -> Product2/1
  Demux/3 -> Product2/2
  Product2/1 -> Add/3
  Product/1 -> Il/1
  "Iabc_o "/1 -> Demux/1

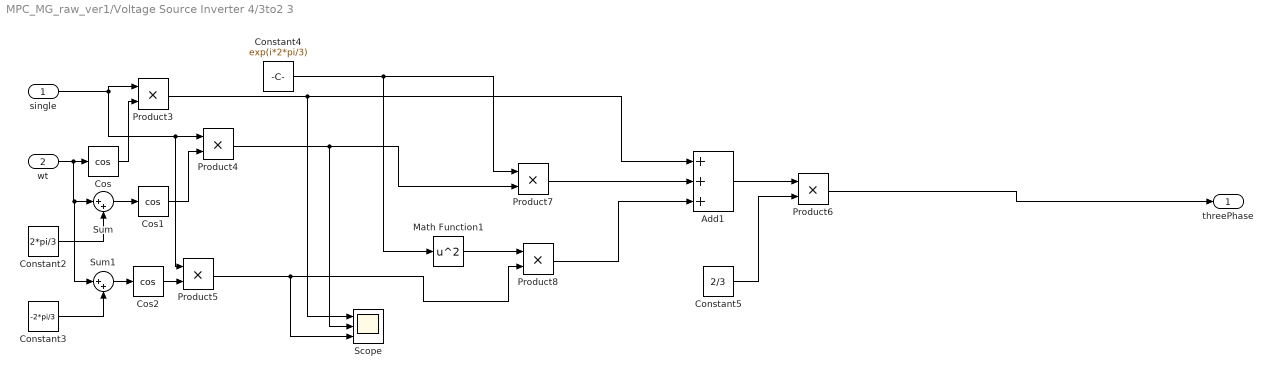
== system MPC_MG_raw_ver1/Voltage Source Inverter 4/3to2 3 ==
  "single " : Inport
  "wt " : Inport  Port=2
  Add1 : Sum  Inputs=+++
  Constant2 : Constant  Value=2*pi/3
  Constant3 : Constant  Value=-2*pi/3
  Constant4 : Constant  Value=exp(i*2*pi/3)
  Constant5 : Constant  Value=2/3
  Cos : Trigonometry  Operator=cos
  Cos1 : Trigonometry  Operator=cos
  Cos2 : Trigonometry  Operator=cos
  Math Function1 : Math  Operator=square  SignedPower=on  SaturateOnIntegerOverflow=on
  Product{3..8} (6 alike) : Product  RndMeth=Zero
  Scope : Scope  NumInputPorts=3
  Sum : Sum  Inputs=|++
  Sum1 : Sum  Inputs=|++
  threePhase : Outport  VectorParamsAs1DForOutWhenUnconnected=off
  wires:
  "single "/1 -> Product5/1, Product4/1, Product3/1
  Cos/1 -> Product3/2
  Constant2/1 -> Sum/2
  Sum/1 -> Cos1/1
  Cos1/1 -> Product4/2
  "wt "/1 -> Sum1/1, Sum/1, Cos/1
  Constant3/1 -> Sum1/2
  Sum1/1 -> Cos2/1
  Cos2/1 -> Product5/2
  Constant4/1 -> Product7/1, Math Function1/1
  Product7/1 -> Add1/2
  Add1/1 -> Product6/1
  Product8/1 -> Add1/3
  Product5/1 -> Scope/3, Product8/2
  Product6/1 -> threePhase/1
  Product3/1 -> Scope/1, Add1/1
  Constant5/1 -> Product6/2
  Product4/1 -> Scope/2, Product7/2
  Math Function1/1 -> Product8/1

== system MPC_MG_raw_ver1/Voltage Source Inverter 4/Droop for secondary control2 ==
  P : Inport
  w_nom : Inport  Port=2
  V_nom : Inport  Port=3
  Q : Inport  Port=4
  Gain4 : Gain  Gain=n_q
  Gain5 : Gain  Gain=m_p
  Integrator : Integrator  WrapState=on  WrappedStateUpperValue=2*pi  WrappedStateLowerValue=0
  Sum1 : Sum  Inputs=|+-
  Sum2 : Sum  Inputs=|+-
  Vref : Outport
  wt : Outport  Port=2
  wo : Outport  Port=3
  wires:
  P/1 -> Gain5/1
  w_nom/1 -> Sum2/1
  Gain5/1 -> Sum2/2
  Sum2/1 -> wo/1, Integrator/1  "w"
  Integrator/1 -> wt/1
  V_nom/1 -> Sum1/1  "Vod_s"
  Gain4/1 -> Sum1/2
  Q/1 -> Gain4/1
  Sum1/1 -> Vref/1  "Vod_s"

== system MPC_MG_raw_ver1/Voltage Source Inverter 4/Low-pass filter ==
  p_hat : Inport
  q_hat : Inport  Port=2
  Low-Pass Filter (Discrete or Continuous) : eeGeneralControl/Low-Pass Filter (Discrete or Continuous)  K=1  T=lo_co  B=inf  A=-inf  init_option=Inherited from block input  x0=0  Ts=-1
  Low-Pass Filter (Discrete or Continuous)1 : eeGeneralControl/Low-Pass Filter (Discrete or Continuous)  K=1  T=lo_co  B=inf  A=-inf  init_option=Inherited from block input  x0=0  Ts=-1
  P : Outport
  Q : Outport  Port=2
  wires:
  q_hat/1 -> Low-Pass Filter (Discrete or Continuous)1/1
  Low-Pass Filter (Discrete or Continuous)1/1 -> Q/1  "Q"
  Low-Pass Filter (Discrete or Continuous)/1 -> P/1  "P"
  p_hat/1 -> Low-Pass Filter (Discrete or Continuous)/1

== system MPC_MG_raw_ver1/Voltage Source Inverter 4/PQ calculator ==
  Vod : Inport
  Voq : Inport  Port=2
  Iod : Inport  Port=3
  Ioq : Inport  Port=4
  Product{,1..3} (4 alike) : Product
  Sum10 : Sum  Inputs=|++
  Sum11 : Sum  Inputs=|+-
  p_hat : Outport
  q_hat : Outport  Port=2
  wires:
  Product3/1 -> Sum11/2
  Product1/1 -> Sum10/2
  Voq/1 -> Product3/1, Product1/1
  Iod/1 -> Product/2, Product3/2
  Product2/1 -> Sum11/1
  Ioq/1 -> Product1/2, Product2/2
  Product/1 -> Sum10/1
  Vod/1 -> Product/1, Product2/1
  Sum11/1 -> q_hat/1  "q_hat"
  Sum10/1 -> p_hat/1  "p_hat"

== system MPC_MG_raw_ver1/Voltage Source Inverter 4/dq converter ==
  Vodq : Inport
  Iodq : Inport  Port=2
  Ildq : Inport  Port=3
  wo : Inport  Port=4
  Demux : Demux  Outputs=2
  Demux1 : Demux  Outputs=2
  Demux4 : Demux  Outputs=2
  Selector1 : Selector  InputPortWidth=3  IndexOptions=Index vector (dialog)  Indices=[1 2]  OutputSizes=1
  Selector2 : Selector  InputPortWidth=3  IndexOptions=Index vector (dialog)  Indices=[1 2]  OutputSizes=1
  Selector3 : Selector  InputPortWidth=3  IndexOptions=Index vector (dialog)  Indices=[1 2]  OutputSizes=1
  abc to dq0 : spsabctodq0Lib/abc to dq0  Alignment=90 degrees behind phase A axis
  abc to dq1 : spsabctodq0Lib/abc to dq0  Alignment=90 degrees behind phase A axis
  abc to dq2 : spsabctodq0Lib/abc to dq0  Alignment=90 degrees behind phase A axis
  Vod : Outport
  Voq : Outport  Port=2
  Iod : Outport  Port=3
  Ioq : Outport  Port=4
  Ild : Outport  Port=5
  Ilq : Outport  Port=6
  wires:
  Vodq/1 -> abc to dq0/1
  Demux/1 -> Vod/1  "Vod"
  Demux1/1 -> Iod/1  "Iod"
  Selector3/1 -> Demux4/1
  Demux/2 -> Voq/1  "Voq"
  Selector1/1 -> Demux/1
  abc to dq2/1 -> Selector2/1
  abc to dq1/1 -> Selector3/1
  wo/1 -> abc to dq0/2, abc to dq2/2, abc to dq1/2
  Demux1/2 -> Ioq/1  "Ioq"
  Demux4/1 -> Ild/1  "Ild"
  abc to dq0/1 -> Selector1/1
  Selector2/1 -> Demux1/1
  Iodq/1 -> abc to dq2/1
  Ildq/1 -> abc to dq1/1
  Demux4/2 -> Ilq/1  "Ilq"

== system MPC_MG_raw_ver1/Voltage Source Inverter 4/remap ==
  In1 : Inport
  Demux : Demux  Outputs=6
  Mux : Mux  Inputs=6
  Out1 : Outport
  wires:
  Demux/5 -> Mux/4
  Demux/3 -> Mux/5
  Demux/2 -> Mux/3
  Demux/4 -> Mux/2
  In1/1 -> Demux/1
  Demux/1 -> Mux/1
  Demux/6 -> Mux/6
  Mux/1 -> Out1/1

== system MPC_MG_raw_ver1/Voltage Source Inverter 5/3to2 1 ==
  "Vabc_o " : Inport
  Add : Sum  Inputs=+++
  Constant : Constant  Value=exp(i*2*pi/3)
  Constant1 : Constant  Value=2/3
  Demux : Demux  Outputs=3
  Math Function : Math  Operator=square  SignedPower=on  SaturateOnIntegerOverflow=on
  Product : Product  RndMeth=Zero
  Product1 : Product  RndMeth=Zero
  Product2 : Product  RndMeth=Zero
  Vo : Outport  VectorParamsAs1DForOutWhenUnconnected=off
  wires:
  Add/1 -> Product/1
  Demux/1 -> Add/1
  Constant1/1 -> Product/2
  Product1/1 -> Add/2
  Constant/1 -> Product1/1, Math Function/1
  Demux/2 -> Product1/2
  Math Function/1 -> Product2/1
  Demux/3 -> Product2/2
  Product2/1 -> Add/3
  Product/1 -> Vo/1
  "Vabc_o "/1 -> Demux/1

== system MPC_MG_raw_ver1/Voltage Source Inverter 5/3to2 2 ==
  "Iabc_o " : Inport
  Add : Sum  Inputs=+++
  Constant : Constant  Value=exp(i*2*pi/3)
  Constant1 : Constant  Value=2/3
  Demux : Demux  Outputs=3
  Math Function : Math  Operator=square  SignedPower=on  SaturateOnIntegerOverflow=on
  Product : Product  RndMeth=Zero
  Product1 : Product  RndMeth=Zero
  Product2 : Product  RndMeth=Zero
  Il : Outport  VectorParamsAs1DForOutWhenUnconnected=off
  wires:
  Add/1 -> Product/1
  Demux/1 -> Add/1
  Constant1/1 -> Product/2
  Product1/1 -> Add/2
  Constant/1 -> Product1/1, Math Function/1
  Demux/2 -> Product1/2
  Math Function/1 -> Product2/1
  Demux/3 -> Product2/2
  Product2/1 -> Add/3
  Product/1 -> Il/1
  "Iabc_o "/1 -> Demux/1

== system MPC_MG_raw_ver1/Voltage Source Inverter 5/3to2 3 ==
  "single " : Inport
  "wt " : Inport  Port=2
  Add1 : Sum  Inputs=+++
  Constant2 : Constant  Value=2*pi/3
  Constant3 : Constant  Value=-2*pi/3
  Constant4 : Constant  Value=exp(i*2*pi/3)
  Constant5 : Constant  Value=2/3
  Cos : Trigonometry  Operator=cos
  Cos1 : Trigonometry  Operator=cos
  Cos2 : Trigonometry  Operator=cos
  Math Function1 : Math  Operator=square  SignedPower=on  SaturateOnIntegerOverflow=on
  Product{3..8} (6 alike) : Product  RndMeth=Zero
  Scope : Scope  NumInputPorts=3
  Sum : Sum  Inputs=|++
  Sum1 : Sum  Inputs=|++
  threePhase : Outport  VectorParamsAs1DForOutWhenUnconnected=off
  wires:
  "single "/1 -> Product5/1, Product4/1, Product3/1
  Cos/1 -> Product3/2
  Constant2/1 -> Sum/2
  Sum/1 -> Cos1/1
  Cos1/1 -> Product4/2
  "wt "/1 -> Sum1/1, Sum/1, Cos/1
  Constant3/1 -> Sum1/2
  Sum1/1 -> Cos2/1
  Cos2/1 -> Product5/2
  Constant4/1 -> Product7/1, Math Function1/1
  Product7/1 -> Add1/2
  Add1/1 -> Product6/1
  Product8/1 -> Add1/3
  Product5/1 -> Scope/3, Product8/2
  Product6/1 -> threePhase/1
  Product3/1 -> Scope/1, Add1/1
  Constant5/1 -> Product6/2
  Product4/1 -> Scope/2, Product7/2
  Math Function1/1 -> Product8/1

== system MPC_MG_raw_ver1/Voltage Source Inverter 5/Droop for secondary control2 ==
  P : Inport
  w_nom : Inport  Port=2
  V_nom : Inport  Port=3
  Q : Inport  Port=4
  Gain4 : Gain  Gain=n_q
  Gain5 : Gain  Gain=m_p
  Integrator : Integrator  WrapState=on  WrappedStateUpperValue=2*pi  WrappedStateLowerValue=0
  Sum1 : Sum  Inputs=|+-
  Sum2 : Sum  Inputs=|+-
  Vref : Outport
  wt : Outport  Port=2
  wo : Outport  Port=3
  wires:
  P/1 -> Gain5/1
  w_nom/1 -> Sum2/1
  Gain5/1 -> Sum2/2
  Sum2/1 -> wo/1, Integrator/1  "w"
  Integrator/1 -> wt/1
  V_nom/1 -> Sum1/1  "Vod_s"
  Gain4/1 -> Sum1/2
  Q/1 -> Gain4/1
  Sum1/1 -> Vref/1  "Vod_s"

== system MPC_MG_raw_ver1/Voltage Source Inverter 5/Low-pass filter ==
  p_hat : Inport
  q_hat : Inport  Port=2
  Low-Pass Filter (Discrete or Continuous) : eeGeneralControl/Low-Pass Filter (Discrete or Continuous)  K=1  T=lo_co  B=inf  A=-inf  init_option=Inherited from block input  x0=0  Ts=-1
  Low-Pass Filter (Discrete or Continuous)1 : eeGeneralControl/Low-Pass Filter (Discrete or Continuous)  K=1  T=lo_co  B=inf  A=-inf  init_option=Inherited from block input  x0=0  Ts=-1
  P : Outport
  Q : Outport  Port=2
  wires:
  q_hat/1 -> Low-Pass Filter (Discrete or Continuous)1/1
  Low-Pass Filter (Discrete or Continuous)1/1 -> Q/1  "Q"
  Low-Pass Filter (Discrete or Continuous)/1 -> P/1  "P"
  p_hat/1 -> Low-Pass Filter (Discrete or Continuous)/1

== system MPC_MG_raw_ver1/Voltage Source Inverter 5/PQ calculator ==
  Vod : Inport
  Voq : Inport  Port=2
  Iod : Inport  Port=3
  Ioq : Inport  Port=4
  Product{,1..3} (4 alike) : Product
  Sum10 : Sum  Inputs=|++
  Sum11 : Sum  Inputs=|+-
  p_hat : Outport
  q_hat : Outport  Port=2
  wires:
  Product3/1 -> Sum11/2
  Product1/1 -> Sum10/2
  Voq/1 -> Product3/1, Product1/1
  Iod/1 -> Product/2, Product3/2
  Product2/1 -> Sum11/1
  Ioq/1 -> Product1/2, Product2/2
  Product/1 -> Sum10/1
  Vod/1 -> Product/1, Product2/1
  Sum11/1 -> q_hat/1  "q_hat"
  Sum10/1 -> p_hat/1  "p_hat"

== system MPC_MG_raw_ver1/Voltage Source Inverter 5/dq converter ==
  Vodq : Inport
  Iodq : Inport  Port=2
  Ildq : Inport  Port=3
  wo : Inport  Port=4
  Demux : Demux  Outputs=2
  Demux1 : Demux  Outputs=2
  Demux4 : Demux  Outputs=2
  Selector1 : Selector  InputPortWidth=3  IndexOptions=Index vector (dialog)  Indices=[1 2]  OutputSizes=1
  Selector2 : Selector  InputPortWidth=3  IndexOptions=Index vector (dialog)  Indices=[1 2]  OutputSizes=1
  Selector3 : Selector  InputPortWidth=3  IndexOptions=Index vector (dialog)  Indices=[1 2]  OutputSizes=1
  abc to dq0 : powerlib_meascontrol/Transformations/abc to dq0  Alignment=90 degrees behind phase A axis
  abc to dq1 : powerlib_meascontrol/Transformations/abc to dq0  Alignment=90 degrees behind phase A axis
  abc to dq2 : powerlib_meascontrol/Transformations/abc to dq0  Alignment=90 degrees behind phase A axis
  Vod : Outport
  Voq : Outport  Port=2
  Iod : Outport  Port=3
  Ioq : Outport  Port=4
  Ild : Outport  Port=5
  Ilq : Outport  Port=6
  wires:
  Vodq/1 -> abc to dq0/1
  Demux/1 -> Vod/1  "Vod"
  Demux1/1 -> Iod/1  "Iod"
  Selector3/1 -> Demux4/1
  Demux/2 -> Voq/1  "Voq"
  Selector1/1 -> Demux/1
  abc to dq2/1 -> Selector2/1
  abc to dq1/1 -> Selector3/1
  wo/1 -> abc to dq0/2, abc to dq2/2, abc to dq1/2
  Demux1/2 -> Ioq/1  "Ioq"
  Demux4/1 -> Ild/1  "Ild"
  abc to dq0/1 -> Selector1/1
  Selector2/1 -> Demux1/1
  Iodq/1 -> abc to dq2/1
  Ildq/1 -> abc to dq1/1
  Demux4/2 -> Ilq/1  "Ilq"

== system MPC_MG_raw_ver1/Voltage Source Inverter 5/remap ==
  In1 : Inport
  Demux : Demux  Outputs=6
  Mux : Mux  Inputs=6
  Out1 : Outport
  wires:
  Demux/5 -> Mux/4
  Demux/3 -> Mux/5
  Demux/2 -> Mux/3
  Demux/4 -> Mux/2
  In1/1 -> Demux/1
  Demux/1 -> Mux/1
  Demux/6 -> Mux/6
  Mux/1 -> Out1/1
